simulink model "Signal_Routing_Lib"  (R2020b)
settings: Solver=VariableStepAuto  StartTime=0.0  StopTime=10.0  RelTol=1e-3
libraries: simulink x8
settings Model: Creator=Emiliano  LastModifiedBy=Emiliano

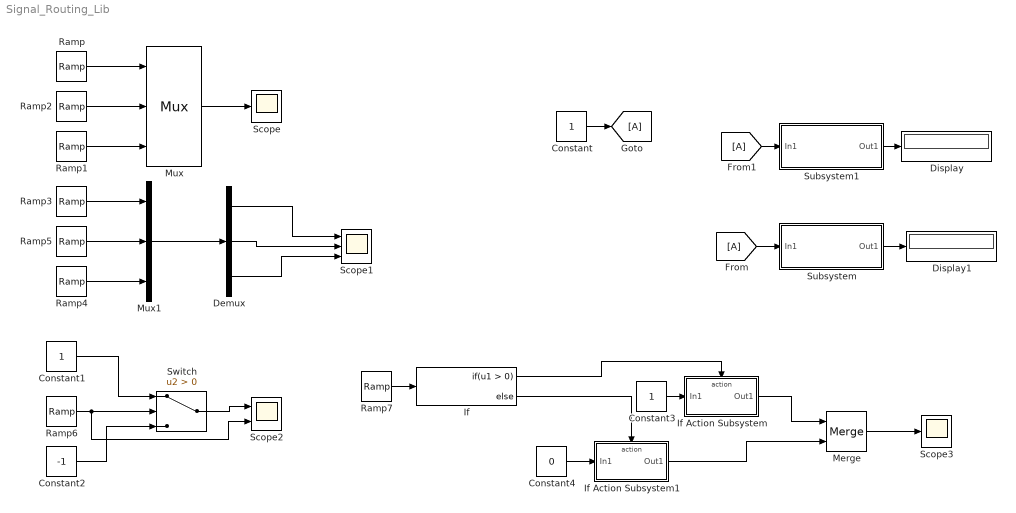
== system Signal_Routing_Lib ==
  Constant : Constant
  Constant1 : Constant
  Constant2 : Constant  Value=-1
  Constant3 : Constant
  Constant4 : Constant  Value=0
  Demux : Demux  Outputs=3
  Display : Display
  Display1 : Display
  If : If
  If Action Subsystem : Subsystem  TreatAsAtomicUnit=on
  If Action Subsystem1 : Subsystem  TreatAsAtomicUnit=on
  Merge : Merge
  Mux : Mux  Inputs=3
      settings: DisplayOption=signals
  Mux1 : Mux  Inputs=3
  Ramp : simulink/Sources/Ramp  slope=2  start=0  InitialOutput=0
  Ramp1 : simulink/Sources/Ramp  slope=0.1  start=0  InitialOutput=0
  Ramp2 : simulink/Sources/Ramp  slope=0.5  start=0  InitialOutput=0
  Ramp3 : simulink/Sources/Ramp  slope=2  start=0  InitialOutput=0
  Ramp4 : simulink/Sources/Ramp  slope=0.1  start=0  InitialOutput=0
  Ramp5 : simulink/Sources/Ramp  slope=0.5  start=0  InitialOutput=0
  Ramp6 : simulink/Sources/Ramp  slope=1  start=0  InitialOutput=-5
  Ramp7 : simulink/Sources/Ramp  slope=1  start=0  InitialOutput=-5
  Scope : Scope
  Scope1 : Scope  NumInputPorts=3
  Scope2 : Scope  NumInputPorts=2
  Scope3 : Scope
  Subsystem : Subsystem
  Subsystem1 : Subsystem
  Switch : Switch  Criteria=u2 > Threshold
  wires:
  Ramp/1 -> Mux/1
  Ramp2/1 -> Mux/2
  Ramp1/1 -> Mux/3
  Mux/1 -> Scope/1
  Ramp5/1 -> Mux1/2
  Ramp4/1 -> Mux1/3
  Ramp3/1 -> Mux1/1
  Mux1/1 -> Demux/1
  Demux/1 -> Scope1/1
  Demux/2 -> Scope1/2
  Demux/3 -> Scope1/3
  Constant/1 -> [A]
  [A] -> Subsystem/1(In1)
  [A] -> Subsystem1/1(In1)
  Subsystem1/1(Out1) -> Display/1
  Subsystem/1(Out1) -> Display1/1
  Constant1/1 -> Switch/1
  Constant2/1 -> Switch/3
  Ramp6/1 -> Switch/2, Scope2/2
  Switch/1 -> Scope2/1
  If/1 -> If Action Subsystem/Action
  If/2 -> If Action Subsystem1/Action
  Constant3/1 -> If Action Subsystem/1(In1)
  Constant4/1 -> If Action Subsystem1/1(In1)
  Ramp7/1 -> If/1
  If Action Subsystem/1(Out1) -> Merge/1
  If Action Subsystem1/1(Out1) -> Merge/2
  Merge/1 -> Scope3/1

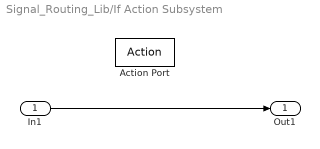
== system Signal_Routing_Lib/If Action Subsystem ==
  In1 : Inport
  Action Port : ActionPort  ActionPortLabel=if(u1 > 0)
  Out1 : Outport
  wires:
  In1/1 -> Out1/1

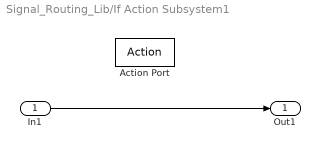
== system Signal_Routing_Lib/If Action Subsystem1 ==
  In1 : Inport
  Action Port : ActionPort  ActionPortLabel=else
  Out1 : Outport
  wires:
  In1/1 -> Out1/1

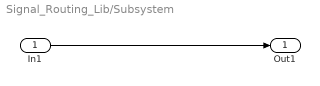
== system Signal_Routing_Lib/Subsystem ==
  In1 : Inport
  Out1 : Outport
  wires:
  In1/1 -> Out1/1

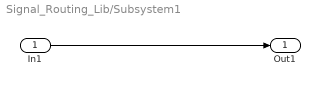
== system Signal_Routing_Lib/Subsystem1 ==
  In1 : Inport
  Out1 : Outport
  wires:
  In1/1 -> Out1/1
